simulink subsystem "RRR_elastic_joints"  (R2021b)
settings: Solver=VariableStepAuto  StartTime=0.0  StopTime=10.0  RelTol=1e-3
undefined symbols (not defined in the file): Im1, Im2, Im3, k, theta0, thetad0
settings Model: Creator=fabioscap  LastModifiedBy=fabioscap

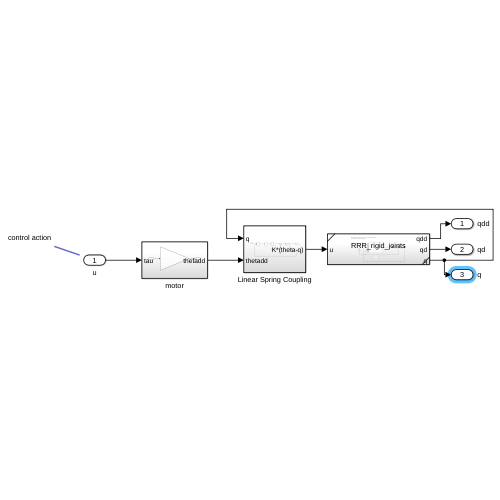
[thumbnail: Simulink's stored preview of the top-level diagram]
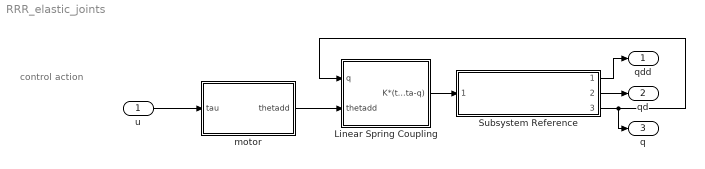
== system RRR_elastic_joints ==
  note: control action
  u : Inport
  Linear Spring Coupling : Subsystem
  Subsystem Reference : Subsystem  ReferencedSubsystem=RRR_rigid_joints
  motor : Subsystem
  qdd : Outport
  qd : Outport  Port=2
  q : Outport  Port=3
  wires:
  motor/1(thetadd) -> Linear Spring Coupling/2(thetadd)
  u/1 -> motor/1(tau)
  Linear Spring Coupling/1(K*(theta-q)) -> Subsystem Reference/1
  Subsystem Reference/1 -> qdd/1
  Subsystem Reference/2 -> qd/1
  Subsystem Reference/3 -> q/1, Linear Spring Coupling/1(q)

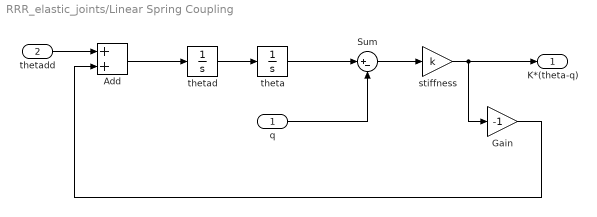
== system RRR_elastic_joints/Linear Spring Coupling ==
  q : Inport  PortDimensions=3
  thetadd : Inport  Port=2  PortDimensions=3
  Add : Sum
  Gain : Gain  Gain=-1
  Sum : Sum  Inputs=|+-
  stiffness : Gain  Gain=k
  theta : Integrator  InitialCondition=theta0
  thetad : Integrator  InitialCondition=thetad0
  K*(theta-q) : Outport
  wires:
  stiffness/1 -> K*(theta-q)/1, Gain/1
  Add/1 -> thetad/1
  thetad/1 -> theta/1
  Gain/1 -> Add/2
  theta/1 -> Sum/1
  Sum/1 -> stiffness/1
  q/1 -> Sum/2
  thetadd/1 -> Add/1

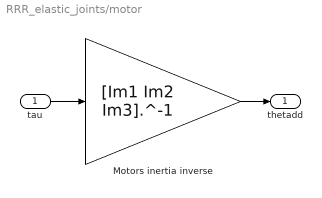
== system RRR_elastic_joints/motor ==
  tau : Inport
  Motors inertia inverse : Gain  Gain=[Im1 Im2 Im3].^-1
  thetadd : Outport
  wires:
  tau/1 -> Motors inertia inverse/1
  Motors inertia inverse/1 -> thetadd/1
